simulink model "sulfitador"  (R2021a)
settings: Solver=ode45  StartTime=0.0  StopTime=2000  MaxStep=10  RelTol=1e-3  AbsTol=1e-3  EnableMultiTasking=on
libraries: fuzblock x1
settings Model: ExtModeTrigMode=oneshot  ExtModeArmWhenConnect=off  Creator=david  LastModifiedBy=david
settings SolverCC: AutoScaleAbsTol=off
settings DataIOCC: SaveFormat=Array  SignalLoggingSaveFormat=ModelDataLogs  SaveOutput=off  SaveTime=off  ReturnWorkspaceOutputs=off
settings OptimizationCC: BlockReduction=off  BooleanDataType=off  InitFltsAndDblsToZero=on  LifeSpan=inf
settings DebuggingCC: SaveWithParameterizedLinksMsg=none  UnderspecifiedInitializationDetection=Classic  MergeDetectMultiDrivingBlocksExec=none  SignalResolutionControl=TryResolveAllWithWarning  MultiTaskDSMMsg=warning  MultiTaskCondExecSysMsg=none  FcnCallInpInsideContextMsg=warning  SFUnexpectedBacktrackingDiag=warning  SFNoUnconditionalDefaultTransitionDiag=warning  SFExecutionAtInitializationDiag=none  SFMachineParentedDataDiag=warning  ArithmeticOperatorsInVariantConditions=warning
settings HardwareCC: ProdBitPerPointer=32  ProdBitPerSizeT=32  ProdBitPerPtrDiffT=32  ProdLargestAtomicFloat=None  ProdIntDivRoundTo=Undefined  ProdEndianess=Unspecified  ProdWordSize=32  ProdHWDeviceType=32-bit Generic  TargetUnknown=on
settings ModelReferenceCC: PropagateSignalLabelsOutOfModel=off
settings CodeAppCC: StateflowObjectComments=on
settings GRTTargetCC: TargetFcnLib=ansi_tfl_tmw.mat  TargetLangStandard=C89/C90 (ANSI)  ModelReferenceCompliant=off  ParMdlRefBuildCompliant=off  CompOptLevelCompliant=off  ConcurrentExecutionCompliant=off  CombineOutputUpdateFcns=off  MatFileLogging=off  MATLABClassNameForMDSCustomization=Simulink.SoftwareTarget.TargetSpecificTriggerConfigurationBase  GRTInterface=on
settings ConfigComp: CovMetricSettings=dw  CovSaveCumulativeToWorkspaceVar=on  CovSaveSingleToWorkspaceVar=on

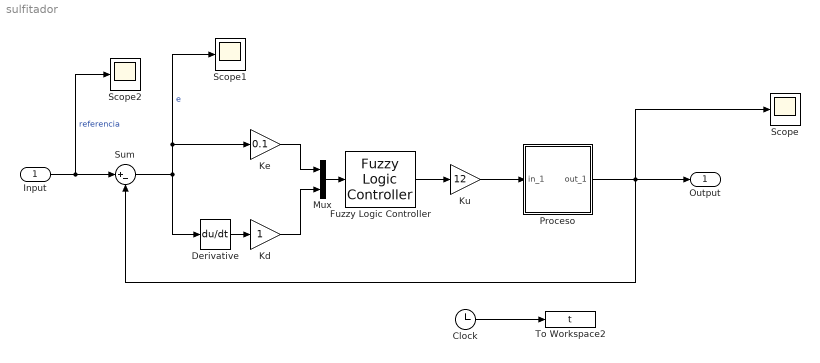
== system sulfitador ==
  Input : Inport
  Clock : Clock
  Derivative : Derivative
  Fuzzy Logic Controller : fuzblock/Fuzzy Logic  Controller  FIS=SulfitadorMandani2022  OutputSampleNumber=101  DataType=double  FuzzifiedInputs=off  RuleFiringStrengths=off  RuleOutputs=off  AggregatedOutputs=off  SimulateUsing=Interpreted execution  OutOfRangeInputValueMessage=warning  NoRuleFiredMessage=warning  EmptyOutputFuzzySetMessage=warning
  Kd : Gain
  Ke : Gain  Gain=0.1
  Ku : Gain  Gain=12
  Mux : Mux  Inputs=2
  Proceso : Subsystem
  Scope : Scope
  Scope1 : Scope
  Scope2 : Scope
  Sum : Sum  Inputs=|+-
  To Workspace2 : ToWorkspace  VariableName=t
      settings: MaxDataPoints=5000
  Output : Outport
  wires:
  Clock/1 -> To Workspace2/1
  Ku/1 -> Proceso/1(in_1)
  Fuzzy Logic Controller/1 -> Ku/1
  Derivative/1 -> Kd/1
  Proceso/1(out_1) -> Output/1, Sum/2, Scope/1
  Sum/1 -> Scope1/1, Ke/1, Derivative/1  "e"
  Input/1 -> Scope2/1, Sum/1  "referencia"
  Mux/1 -> Fuzzy Logic Controller/1
  Ke/1 -> Mux/1
  Kd/1 -> Mux/2

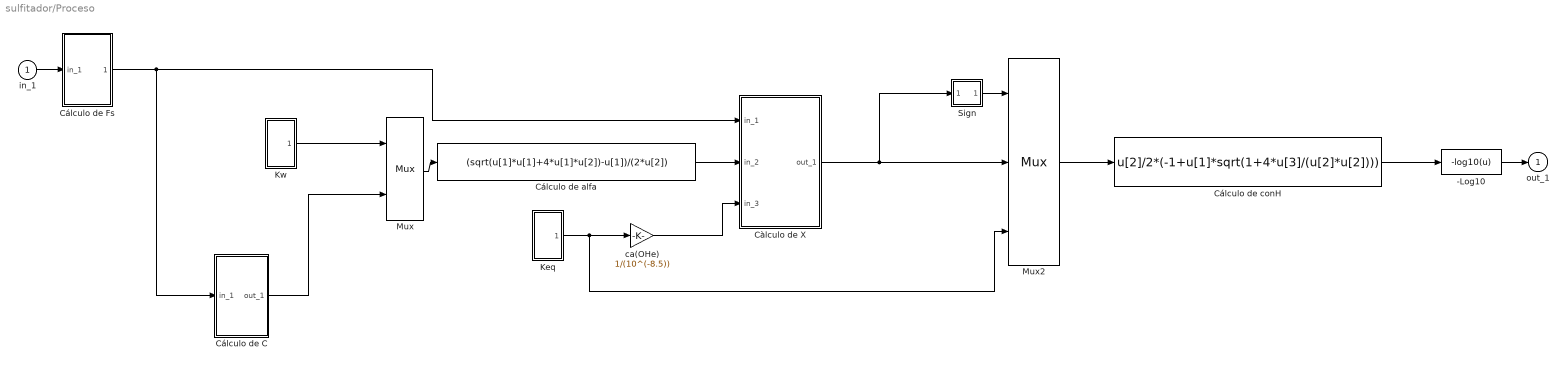
== system sulfitador/Proceso ==
  in_1 : Inport
  "-Log10 " : Fcn  Expr=-log10(u)
  Càlculo de X : Subsystem
  Cálculo de C : Subsystem
  "Cálculo de Fs " : Subsystem
  Cálculo de alfa : Fcn  Expr=(sqrt(u[1]*u[1]+4*u[1]*u[2])-u[1])/(2*u[2])
  "Cálculo de conH " : Fcn  Expr=u[2]/2*(-1+u[1]*sqrt(1+4*u[3]/(u[2]*u[2])))
  Keq : Subsystem
  "Kw " : Subsystem
  Mux : Mux  Inputs=2
  Mux2 : Mux  Inputs=3
  Sign : Subsystem  mask(Sign){}
      mask help: y = sign(x)
      mask Help: Sign Function:\n\t\t\ty = 1 if x > 0\n\t\t\ty = 0 if x = 0\n\t\t\ty = -1 if x < 0
      mask Display: plot(-50,-50,50,50,[-50,50],[0,0],[0,0],[-50,50],[-40,0],[-30,-30],[0,40],[30,30])
  ca(OHe) : Gain  Gain=1/(10^(-8.5))  SaturateOnIntegerOverflow=on  OutDataTypeStr=Inherit: Same as input  ParamDataTypeStr=Inherit: Same as input
  out_1 : Outport
  wires:
  Cálculo de alfa/1 -> Càlculo de X/2(in_2)
  Mux/1 -> Cálculo de alfa/1
  Sign/1(out_1) -> Mux2/1
  "Cálculo de conH "/1 -> "-Log10 "/1
  Mux2/1 -> "Cálculo de conH "/1
  in_1/1 -> "Cálculo de Fs "/1(in_1)
  "-Log10 "/1 -> out_1/1
  Càlculo de X/1(out_1) -> Mux2/2, Sign/1(in_1)
  Cálculo de C/1(out_1) -> Mux/2
  "Kw "/1(out_1) -> Mux/1
  "Cálculo de Fs "/1(out_1) -> Càlculo de X/1(in_1), Cálculo de C/1(in_1)
  ca(OHe)/1 -> Càlculo de X/3(in_3)
  Keq/1(out_1) -> ca(OHe)/1, Mux2/3

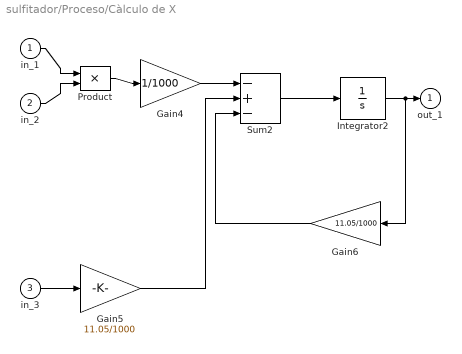
== system sulfitador/Proceso/Càlculo de X ==
  in_1 : Inport
  in_2 : Inport  Port=2
  in_3 : Inport  Port=3
  Gain4 : Gain  Gain=1/1000  SaturateOnIntegerOverflow=on  OutDataTypeStr=Inherit: Same as input  ParamDataTypeStr=Inherit: Same as input
  Gain5 : Gain  Gain=11.05/1000  SaturateOnIntegerOverflow=on  OutDataTypeStr=Inherit: Same as input  ParamDataTypeStr=Inherit: Same as input
  Gain6 : Gain  Gain=11.05/1000  SaturateOnIntegerOverflow=on  OutDataTypeStr=Inherit: Same as input  ParamDataTypeStr=Inherit: Same as input
  Integrator2 : Integrator  InitialCondition=-3.1315e-6
  Product : Product  InputSameDT=on  RndMeth=Zero  SaturateOnIntegerOverflow=on  OutDataTypeStr=Inherit: Same as first input
  Sum2 : Sum  Inputs=-+-  InputSameDT=on  SaturateOnIntegerOverflow=on  OutDataTypeStr=Inherit: Same as first input
  out_1 : Outport
  wires:
  Gain5/1 -> Sum2/2
  Gain6/1 -> Sum2/3
  Sum2/1 -> Integrator2/1
  Gain4/1 -> Sum2/1
  Product/1 -> Gain4/1
  in_1/1 -> Product/1
  in_2/1 -> Product/2
  Integrator2/1 -> Gain6/1, out_1/1
  in_3/1 -> Gain5/1

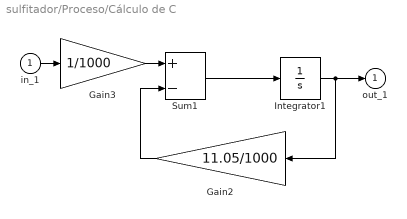
== system sulfitador/Proceso/Cálculo de C ==
  in_1 : Inport
  Gain2 : Gain  Gain=11.05/1000  SaturateOnIntegerOverflow=on  OutDataTypeStr=Inherit: Same as input  ParamDataTypeStr=Inherit: Same as input
  Gain3 : Gain  Gain=1/1000  SaturateOnIntegerOverflow=on  OutDataTypeStr=Inherit: Same as input  ParamDataTypeStr=Inherit: Same as input
  Integrator1 : Integrator  InitialCondition=0.9*0.1652/11.05
  Sum1 : Sum  Inputs=+-  InputSameDT=on  SaturateOnIntegerOverflow=on  OutDataTypeStr=Inherit: Same as first input
  out_1 : Outport
  wires:
  Gain2/1 -> Sum1/2
  Sum1/1 -> Integrator1/1
  Gain3/1 -> Sum1/1
  in_1/1 -> Gain3/1
  Integrator1/1 -> Gain2/1, out_1/1

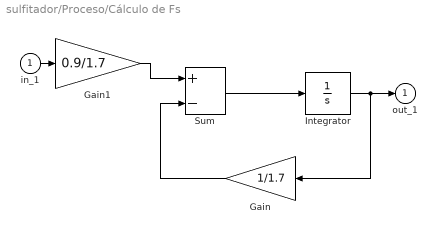
== system sulfitador/Proceso/Cálculo de Fs  ==
  in_1 : Inport
  Gain : Gain  Gain=1/1.7  SaturateOnIntegerOverflow=on  OutDataTypeStr=Inherit: Same as input  ParamDataTypeStr=Inherit: Same as input
  Gain1 : Gain  Gain=0.9/1.7  SaturateOnIntegerOverflow=on  OutDataTypeStr=Inherit: Same as input  ParamDataTypeStr=Inherit: Same as input
  Integrator : Integrator  InitialCondition=0.9*0.1652
  Sum : Sum  Inputs=+-  InputSameDT=on  SaturateOnIntegerOverflow=on  OutDataTypeStr=Inherit: Same as first input
  out_1 : Outport
  wires:
  Gain/1 -> Sum/2
  Sum/1 -> Integrator/1
  Gain1/1 -> Sum/1
  in_1/1 -> Gain1/1
  Integrator/1 -> Gain/1, out_1/1

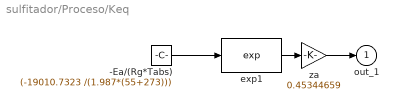
== system sulfitador/Proceso/Keq ==
  -Ea/(Rg*Tabs) : Constant  Value=(-19010.7323 /(1.987*(55+273)))
  exp1 : MATLABFcn  MATLABFcn=exp
  "za " : Gain  Gain=0.45344659  SaturateOnIntegerOverflow=on  OutDataTypeStr=Inherit: Same as input  ParamDataTypeStr=Inherit: Same as input
  out_1 : Outport
  wires:
  exp1/1 -> "za "/1
  -Ea/(Rg*Tabs)/1 -> exp1/1
  "za "/1 -> out_1/1

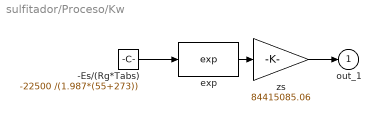
== system sulfitador/Proceso/Kw  ==
  -Es/(Rg*Tabs) : Constant  Value=-22500 /(1.987*(55+273))
  exp : MATLABFcn  MATLABFcn=exp
  zs : Gain  Gain=84415085.06  SaturateOnIntegerOverflow=on  OutDataTypeStr=Inherit: Same as input  ParamDataTypeStr=Inherit: Same as input
  out_1 : Outport
  wires:
  exp/1 -> zs/1
  -Es/(Rg*Tabs)/1 -> exp/1
  zs/1 -> out_1/1

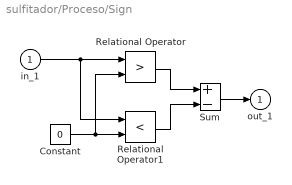
== system sulfitador/Proceso/Sign ==
  in_1 : Inport
  Constant : Constant  Value=0
  Relational Operator : RelationalOperator  Operator=>  RndMeth=Nearest  InputSameDT=on
  Relational Operator1 : RelationalOperator  Operator=<  RndMeth=Nearest  InputSameDT=on
  Sum : Sum  Inputs=+-  InputSameDT=on  SaturateOnIntegerOverflow=on  OutDataTypeStr=Inherit: Same as first input
  out_1 : Outport
  wires:
  in_1/1 -> Relational Operator/1, Relational Operator1/1
  Constant/1 -> Relational Operator1/2, Relational Operator/2
  Relational Operator1/1 -> Sum/2
  Relational Operator/1 -> Sum/1
  Sum/1 -> out_1/1
